simulink model "DrvDem"  (R2020b)
settings: configuration reference "cs_ert" (kept outside this file)
settings Model: DataDictionary=DrvDem.sldd  EnableAccessToBaseWorkspace=off  Creator=zhoutinglin  LastModifiedBy=zhoutinglin
settings ConfigSetRef: SourceName=cs_ert

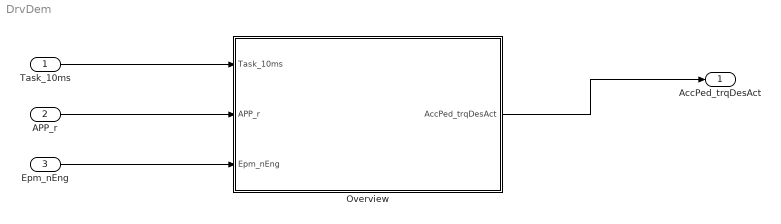
== system DrvDem ==
  Task_10ms : Inport  OutputFunctionCall=on
  APP_r : Inport  Port=2
  Epm_nEng : Inport  Port=3
  Overview : Subsystem
  AccPed_trqDesAct : Outport
  wires:
  Task_10ms/1 -> Overview/1(Task_10ms)
  APP_r/1 -> Overview/2(APP_r)
  Epm_nEng/1 -> Overview/3(Epm_nEng)
  Overview/1(AccPed_trqDesAct) -> AccPed_trqDesAct/1

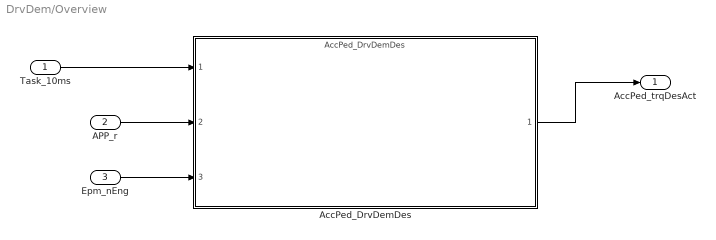
== system DrvDem/Overview ==
  Task_10ms : Inport
  APP_r : Inport  Port=2
  Epm_nEng : Inport  Port=3
  AccPed_DrvDemDes : ModelReference  ModelNameDialog=AccPed_DrvDemDes  SimulationMode=Normal  ScheduleRates=on  ModelReferenceVersion=1.57
  AccPed_trqDesAct : Outport
  wires:
  APP_r/1 -> AccPed_DrvDemDes/2
  Epm_nEng/1 -> AccPed_DrvDemDes/3
  AccPed_DrvDemDes/1 -> AccPed_trqDesAct/1
  Task_10ms/1 -> AccPed_DrvDemDes/1
